simulink model "SixDof"  (R2023a)
settings: Solver=VariableStepAuto  StartTime=0.0  StopTime=60  RelTol=1e-3
values from neighbouring files (symbols this model uses):
  b = 9.144    [FS.m]
  c = 3.45    [FS.m]
  delta_r = 0    [FS.m]
  deltalef = 0    [FS.m]
  deltaSB = 0    [FS.m]
  F16_LookupTables =     [F16_LookupTables.mat]
  g = 9.80665    [FS.m]
  Ixx = 12875    [FS.m]
  Ixz = 1331    [FS.m]
  Iyy = 75674    [FS.m]
  Izz = 85552    [FS.m]
  mass = 9300    [FS.m]
  S = 27.88    [FS.m]
undefined symbols (not defined in the file or in its folder): Earth, WGS84
libraries: coeff x6, simulink_extras x4, shared6dof x1, aerolibtransform2 x1, aerolibfltsims x1, AtmosferModel x1, aerolibasang x1, simulink x1, sharedtransform x1, propulsive x1, uavutilslib x1
(part 2 of 2)

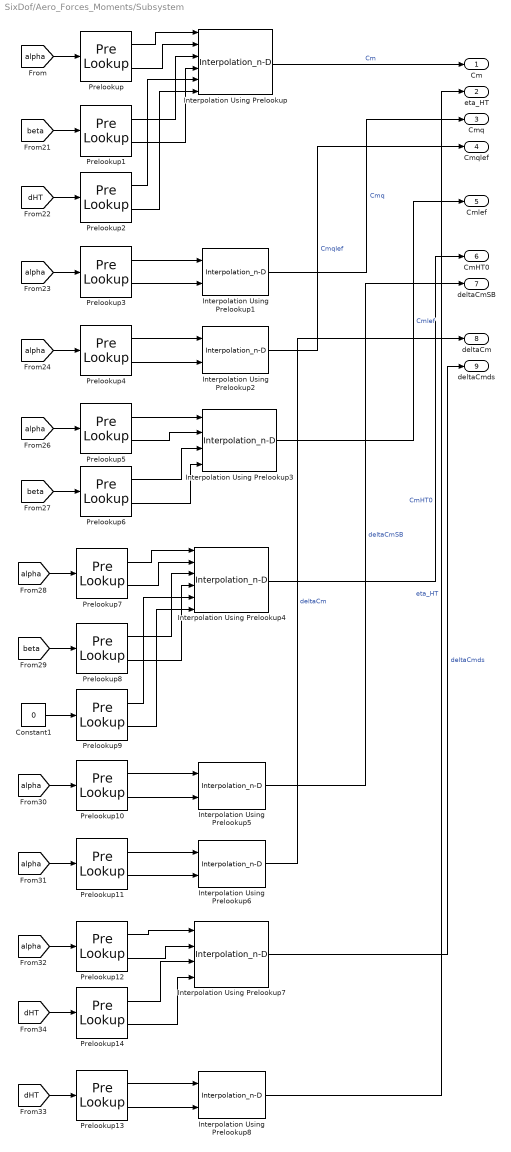
== system SixDof/Aero_Forces_Moments/Subsystem ==
  Constant1 : Constant  Value=0
  Interpolation Using Prelookup : Interpolation_n-D  NumberOfTableDimensions=3  Table=F16_LookupTables.aero.data.Cm.Cm  InternalRulePriority=Speed
      settings: InputPortMap=u0,u1,u2,u3,u4,u5
  Interpolation Using Prelookup1 : Interpolation_n-D  NumberOfTableDimensions=1  Table=F16_LookupTables.aero.data.Cm.Cmq  InternalRulePriority=Speed
      settings: InputPortMap=u0,u1
  Interpolation Using Prelookup2 : Interpolation_n-D  NumberOfTableDimensions=1  Table=F16_LookupTables.aero.data.Cm.deltaCmqlef  InternalRulePriority=Speed
      settings: InputPortMap=u0,u1
  Interpolation Using Prelookup3 : Interpolation_n-D  Table=F16_LookupTables.aero.data.Cm.Cmlef  InternalRulePriority=Speed
  Interpolation Using Prelookup4 : Interpolation_n-D  NumberOfTableDimensions=3  Table=F16_LookupTables.aero.data.Cm.Cm  InternalRulePriority=Speed
      settings: InputPortMap=u0,u1,u2,u3,u4,u5
  Interpolation Using Prelookup5 : Interpolation_n-D  NumberOfTableDimensions=1  Table=F16_LookupTables.aero.data.Cm.deltaCmSB  InternalRulePriority=Speed
      settings: InputPortMap=u0,u1
  Interpolation Using Prelookup6 : Interpolation_n-D  NumberOfTableDimensions=1  Table=F16_LookupTables.aero.data.Cm.deltaCm  InternalRulePriority=Speed
      settings: InputPortMap=u0,u1
  Interpolation Using Prelookup7 : Interpolation_n-D  Table=F16_LookupTables.aero.data.Cm.deltaCmds  InternalRulePriority=Speed
  Interpolation Using Prelookup8 : Interpolation_n-D  NumberOfTableDimensions=1  Table=F16_LookupTables.aero.data.Cm.eta_HT  InternalRulePriority=Speed
      settings: InputPortMap=u0,u1
  Prelookup : PreLookup  BreakpointsData=F16_LookupTables.aero.inputs.Cm.Cm.alpha  ExtrapMethod=Linear
  Prelookup1 : PreLookup  BreakpointsData=F16_LookupTables.aero.inputs.Cm.Cm.beta  ExtrapMethod=Linear
  Prelookup10 : PreLookup  BreakpointsData=F16_LookupTables.aero.inputs.Cm.deltaCmSB.alpha  ExtrapMethod=Linear
  Prelookup11 : PreLookup  BreakpointsData=F16_LookupTables.aero.inputs.Cm.deltaCm.alpha  ExtrapMethod=Linear
  Prelookup12 : PreLookup  BreakpointsData=F16_LookupTables.aero.inputs.Cm.deltaCmds.alpha  ExtrapMethod=Linear
  Prelookup13 : PreLookup  BreakpointsData=F16_LookupTables.aero.inputs.Cm.n_dHT.dHT  ExtrapMethod=Linear
  Prelookup14 : PreLookup  BreakpointsData=F16_LookupTables.aero.inputs.Cm.deltaCmds.dHT  ExtrapMethod=Linear
  Prelookup2 : PreLookup  BreakpointsData=F16_LookupTables.aero.inputs.Cm.Cm.dHT  ExtrapMethod=Linear
  Prelookup3 : PreLookup  BreakpointsData=F16_LookupTables.aero.inputs.Cm.Cmq.alpha  ExtrapMethod=Linear
  Prelookup4 : PreLookup  BreakpointsData=F16_LookupTables.aero.inputs.Cm.deltaCmqlef.alpha  ExtrapMethod=Linear
  Prelookup5 : PreLookup  BreakpointsData=F16_LookupTables.aero.inputs.Cm.Cmlef.alpha  ExtrapMethod=Linear
  Prelookup6 : PreLookup  BreakpointsData=F16_LookupTables.aero.inputs.Cm.Cmlef.beta  ExtrapMethod=Linear
  Prelookup7 : PreLookup  BreakpointsData=F16_LookupTables.aero.inputs.Cm.Cm.alpha  ExtrapMethod=Linear
  Prelookup8 : PreLookup  BreakpointsData=F16_LookupTables.aero.inputs.Cm.Cm.beta  ExtrapMethod=Linear
  Prelookup9 : PreLookup  BreakpointsData=F16_LookupTables.aero.inputs.Cm.Cm.dHT  ExtrapMethod=Linear
  Cm : Outport
  eta_HT : Outport  Port=2
  Cmq : Outport  Port=3
  Cmqlef : Outport  Port=4
  Cmlef : Outport  Port=5
  CmHT0 : Outport  Port=6
  deltaCmSB : Outport  Port=7
  deltaCm : Outport  Port=8
  deltaCmds : Outport  Port=9
  wires:
  Prelookup3/1 -> Interpolation Using Prelookup1/1
  [alpha] -> Prelookup11/1
  [alpha] -> Prelookup5/1
  Prelookup11/1 -> Interpolation Using Prelookup6/1
  [beta] -> Prelookup1/1
  Prelookup/1 -> Interpolation Using Prelookup/1
  [alpha] -> Prelookup12/1
  Prelookup4/1 -> Interpolation Using Prelookup2/1
  Prelookup5/2 -> Interpolation Using Prelookup3/2
  Prelookup11/2 -> Interpolation Using Prelookup6/2
  [beta] -> Prelookup6/1
  Interpolation Using Prelookup7/1 -> deltaCmds/1  "deltaCmds"
  Prelookup4/2 -> Interpolation Using Prelookup2/2
  Prelookup7/2 -> Interpolation Using Prelookup4/2
  [alpha] -> Prelookup4/1
  Prelookup8/2 -> Interpolation Using Prelookup4/4
  Interpolation Using Prelookup6/1 -> deltaCm/1  "deltaCm"
  Prelookup6/2 -> Interpolation Using Prelookup3/4
  Prelookup9/2 -> Interpolation Using Prelookup4/6
  Interpolation Using Prelookup5/1 -> deltaCmSB/1  "deltaCmSB"
  Prelookup5/1 -> Interpolation Using Prelookup3/1
  [dHT] -> Prelookup2/1
  Prelookup/2 -> Interpolation Using Prelookup/2
  Prelookup13/2 -> Interpolation Using Prelookup8/2
  [alpha] -> Prelookup/1
  Interpolation Using Prelookup2/1 -> Cmqlef/1  "Cmqlef"
  [beta] -> Prelookup8/1
  Prelookup2/1 -> Interpolation Using Prelookup/5
  Interpolation Using Prelookup1/1 -> Cmq/1  "Cmq"
  Prelookup6/1 -> Interpolation Using Prelookup3/3
  Prelookup1/1 -> Interpolation Using Prelookup/3
  Prelookup2/2 -> Interpolation Using Prelookup/6
  Prelookup1/2 -> Interpolation Using Prelookup/4
  [dHT] -> Prelookup14/1
  Interpolation Using Prelookup/1 -> Cm/1  "Cm"
  Prelookup12/1 -> Interpolation Using Prelookup7/1
  [alpha] -> Prelookup10/1
  Prelookup12/2 -> Interpolation Using Prelookup7/2
  Prelookup13/1 -> Interpolation Using Prelookup8/1
  [dHT] -> Prelookup13/1
  Prelookup10/1 -> Interpolation Using Prelookup5/1
  Constant1/1 -> Prelookup9/1
  Prelookup14/1 -> Interpolation Using Prelookup7/3
  [alpha] -> Prelookup3/1
  Prelookup3/2 -> Interpolation Using Prelookup1/2
  Interpolation Using Prelookup8/1 -> eta_HT/1  "eta_HT"
  Prelookup9/1 -> Interpolation Using Prelookup4/5
  [alpha] -> Prelookup7/1
  Prelookup14/2 -> Interpolation Using Prelookup7/4
  Prelookup7/1 -> Interpolation Using Prelookup4/1
  Prelookup10/2 -> Interpolation Using Prelookup5/2
  Prelookup8/1 -> Interpolation Using Prelookup4/3
  Interpolation Using Prelookup3/1 -> Cmlef/1  "Cmlef"
  Interpolation Using Prelookup4/1 -> CmHT0/1  "CmHT0"

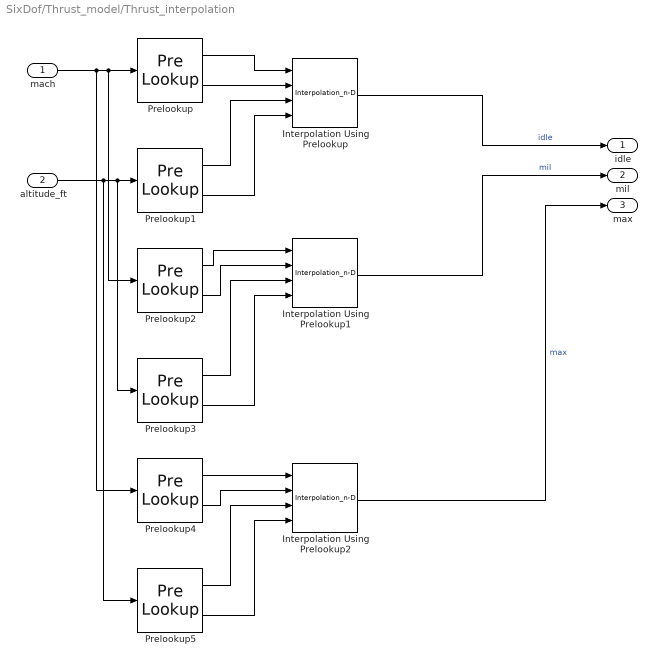
== system SixDof/Thrust_model/Thrust_interpolation ==
  mach : Inport
  altitude_ft : Inport  Port=2
  Interpolation Using Prelookup : Interpolation_n-D  Table=F16_LookupTables.engine.data.Thrust_lbs.idle  InternalRulePriority=Speed
  Interpolation Using Prelookup1 : Interpolation_n-D  Table=F16_LookupTables.engine.data.Thrust_lbs.mil  InternalRulePriority=Speed
  Interpolation Using Prelookup2 : Interpolation_n-D  Table=F16_LookupTables.engine.data.Thrust_lbs.max  InternalRulePriority=Speed
  Prelookup : PreLookup  BreakpointsData=F16_LookupTables.engine.inputs.idle.mach  ExtrapMethod=Linear
  Prelookup1 : PreLookup  BreakpointsData=F16_LookupTables.engine.inputs.idle.alt_ft  ExtrapMethod=Linear
  Prelookup2 : PreLookup  BreakpointsData=F16_LookupTables.engine.inputs.mil.mach  ExtrapMethod=Linear
  Prelookup3 : PreLookup  BreakpointsData=F16_LookupTables.engine.inputs.mil.alt_ft  ExtrapMethod=Linear
  Prelookup4 : PreLookup  BreakpointsData=F16_LookupTables.engine.inputs.max.mach  ExtrapMethod=Linear
  Prelookup5 : PreLookup  BreakpointsData=F16_LookupTables.engine.inputs.max.alt_ft  ExtrapMethod=Linear
  idle : Outport
  mil : Outport  Port=2
  max : Outport  Port=3
  wires:
  Prelookup2/1 -> Interpolation Using Prelookup1/1
  altitude_ft/1 -> Prelookup5/1, Prelookup3/1, Prelookup1/1
  Prelookup1/2 -> Interpolation Using Prelookup/4
  Prelookup5/2 -> Interpolation Using Prelookup2/4
  Prelookup2/2 -> Interpolation Using Prelookup1/2
  Prelookup5/1 -> Interpolation Using Prelookup2/3
  mach/1 -> Prelookup4/1, Prelookup2/1, Prelookup/1
  Prelookup4/1 -> Interpolation Using Prelookup2/1
  Prelookup4/2 -> Interpolation Using Prelookup2/2
  Prelookup/2 -> Interpolation Using Prelookup/2
  Prelookup1/1 -> Interpolation Using Prelookup/3
  Prelookup/1 -> Interpolation Using Prelookup/1
  Prelookup3/1 -> Interpolation Using Prelookup1/3
  Prelookup3/2 -> Interpolation Using Prelookup1/4
  Interpolation Using Prelookup1/1 -> mil/1  "mil"
  Interpolation Using Prelookup/1 -> idle/1  "idle"
  Interpolation Using Prelookup2/1 -> max/1  "max"
